simulink library "library_test"  (R2017b)
settings: Solver=VariableStepAuto  StartTime=0.0  StopTime=10.0  RelTol=1e-3
settings Model: Creator=hbourbou  LastModifiedBy=hbourbou

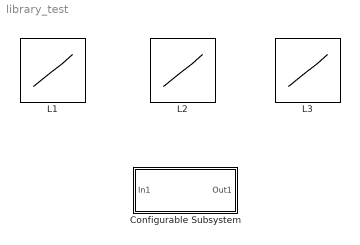
== system library_test ==
  Configurable Subsystem : Subsystem  BlockChoice=L1
      settings: TemplateBlock=self  MemberBlocks=L1,L2,L3
  L1 : Lookup_n-D  NumberOfTableDimensions=1  BreakpointsForDimension1=[-5:5]  Table=tanh([-5:5])  InternalRulePriority=Speed  RndMeth=Simplest  InputSameDT=on
  L2 : Lookup_n-D  NumberOfTableDimensions=1  BreakpointsForDimension1=[-5:5]  Table=cos([-5:5])  InternalRulePriority=Speed  RndMeth=Simplest  InputSameDT=on
  L3 : Lookup_n-D  NumberOfTableDimensions=1  BreakpointsForDimension1=[-5:5]  Table=sin([-5:5])  InternalRulePriority=Speed  RndMeth=Simplest  InputSameDT=on

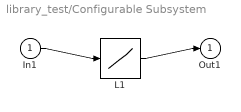
== system library_test/Configurable Subsystem ==
  In1 : Inport
  L1 : Lookup_n-D  NumberOfTableDimensions=1  BreakpointsForDimension1=[-5:5]  Table=tanh([-5:5])  InternalRulePriority=Speed  RndMeth=Simplest  InputSameDT=on
  Out1 : Outport
  wires:
  In1/1 -> L1/1
  L1/1 -> Out1/1
